simulink model "Grid_PBFORCAPF_ab_Detail_2013b_616"  (R2021b)
settings: Solver=FixedStepDiscrete  StartTime=0.0  StopTime=1.5  FixedStep=Ts_Power  RelTol=1e-3
InitFcn:
  | %% Sys Para
  | N=200;fg=50;Vbase=200;
  | Ts_Control=1/N/fg;
  | Tscon=Ts_Control;
  | Ts_Power=Ts_Control/128;
  | fsw=1/Ts_Control;
  | Vdcref=350;
  | Vdcini=Vdcref;
  | 
  | 
  | 
  | %% Load Side
  | Ll=2.0e-3;Rl=1e-2;
  | RL=100;
  | 
  | %% DG Circuit Parameters
  | %% LCL
  | L1_DG1=1.4e-3;R1=1e-3;
  | L2_DG1=0.4e-3;R2=1e-3;
  | Cx_DG1=6.3e-6;
  | 
  | L1_DG2=L1_DG1;L2_DG2=L2_DG1;Cx_DG2=Cx_DG1;
  | L1_DG3=L1_DG1;L2_DG3=L2_DG1;Cx_DG3=Cx_DG1;
  | Cdc=0.55e-3;
  | %PLL;
  | Kp_pll=88;
  | Ki_pll=0.4/Ts_Control;
  | 
  | %% DG2 Controller Parameters
  | Kpc_DG1=4.89;
  | Kic_DG1=0;
  | 
  | Kpdc_DG1=0.2;
  | Kidc_DG1=0.1;
undefined symbols (not defined in the file or in its folder): DiscIntNeverNeededParam, L2, Rd
libraries: spsThreePhaseSeriesRLCBranchLib x13, slpidlib x8, spsThreePhaseVIMeasurementLib x8, spsStairGeneratorLib x8, simulink x6, simulink_extras x6, spsSeriesRLCBranchLib x5, spsThreePhaseBreakerLib x5, spsUniversalBridgeLib x4, spsNeutralLib x4, spsGroundLib x3, spsPWMGenerator2LevelLib x3
(part 1 of 3)
Description:
  | Copyright 2008-2009 The MathWorks(TM), Inc.
settings Model: Creator=hyp01  LastModifiedBy=12586
settings SolverCC: MaxConsecutiveZCs=50000  AlgebraicLoopSolver=TrustRegion  SolverResetMethod=Robust
settings DataIOCC: SaveFormat=Array  SaveOutput=off  SaveTime=off  ReturnWorkspaceOutputs=off  SignalLoggingName=sigsOut
settings OptimizationCC: BlockReduction=off  BooleanDataType=off  ExpressionDepthLimit=2147483647  InitFltsAndDblsToZero=on  LifeSpan=inf
settings DebuggingCC: UnderspecifiedInitializationDetection=Classic  MergeDetectMultiDrivingBlocksExec=none  CheckExecutionContextPreStartOutputMsg=on  SignalResolutionControl=TryResolveAllWithWarning  MaxConsecutiveZCsMsg=none  MultiTaskDSMMsg=warning  MultiTaskCondExecSysMsg=none  FcnCallInpInsideContextMsg=warning  StateNameClashWarn=warning  SFUnexpectedBacktrackingDiag=warning  SFNoUnconditionalDefaultTransitionDiag=warning  SFExecutionAtInitializationDiag=none  SFMachineParentedDataDiag=warning  ArithmeticOperatorsInVariantConditions=warning
settings HardwareCC: ProdBitPerPointer=32  ProdBitPerSizeT=32  ProdBitPerPtrDiffT=32  ProdLargestAtomicFloat=None  ProdIntDivRoundTo=Undefined  ProdEndianess=Unspecified  ProdWordSize=32  ProdHWDeviceType=32-bit Generic  TargetBitPerPointer=64  TargetBitPerSizeT=64  TargetBitPerPtrDiffT=64  TargetLongLongMode=on  TargetIntDivRoundTo=Zero  TargetEndianess=LittleEndian  TargetWordSize=64  TargetHWDeviceType=MATLAB Host  ProdEqTarget=off
settings ModelReferenceCC: PropagateSignalLabelsOutOfModel=off
settings SFSimCC: SimUseLocalCustomCode=off  CustomCodeUndefinedFunction=UseInterfaceOnly
settings RTWCC: RTWUseLocalCustomCode=off  DLArmComputeVersion=20.02.1
settings CodeAppCC: StateflowObjectComments=on
settings GRTTargetCC: TargetFcnLib=ansi_tfl_tmw.mat  TargetLangStandard=C89/C90 (ANSI)  CombineOutputUpdateFcns=off  GRTInterface=on
settings ConfigComp: CovMetricSettings=dw  CovSaveCumulativeToWorkspaceVar=on  CovSaveSingleToWorkspaceVar=on  CovExternalEMLEnable=off
settings SimscapeCC: SimscapeNormalizeSystem=off

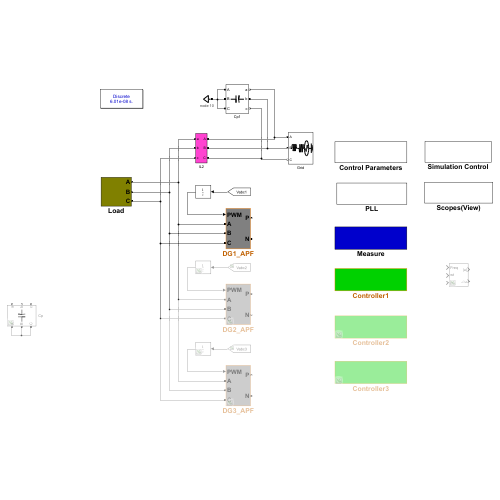
[thumbnail: Simulink's stored preview of the top-level diagram]
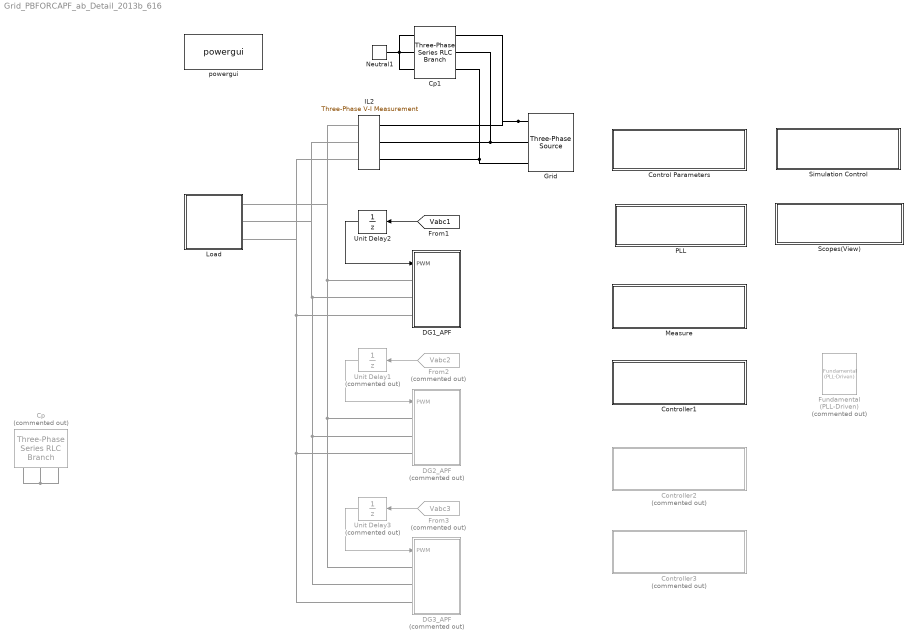
== system Grid_PBFORCAPF_ab_Detail_2013b_616 ==
  Control Parameters : Subsystem
  Controller1 : Subsystem
  Controller2 : Subsystem  Commented=on
  Controller3 : Subsystem  Commented=on
  Cp : spsThreePhaseSeriesRLCBranchLib/Three-Phase Series RLC Branch  Commented=on  LConnTagsString=A|B|C  RConnTagsString=A|B|C  BranchType=C  Resistance=Rd  Inductance=L2  Capacitance=22e-6  Measurements=Branch currents
  Cp1 : spsThreePhaseSeriesRLCBranchLib/Three-Phase Series RLC Branch  LConnTagsString=A|B|C  RConnTagsString=A|B|C  BranchType=C  Resistance=Rd  Inductance=L2  Capacitance=22e-6  Measurements=Branch currents
  DG1_APF : Subsystem
  DG2_APF : Subsystem  Commented=on
  DG3_APF : Subsystem  Commented=on
  From2 : From  Commented=on  GotoTag=Vabc2  TagVisibility=global
      settings: CloseFcn=tagdialog Close
  From3 : From  Commented=on  GotoTag=Vabc3  TagVisibility=global
      settings: CloseFcn=tagdialog Close
  Fundamental (PLL-Driven) : spsFundamentalPLLDrivenLib/Fundamental (PLL-Driven)  Commented=on  Finit=60  Fmin=45  InInit=[1, 0]  Ts=0
      settings: SourceProductBaseCode=PS
  Grid : spsThreePhaseSourceLib/Three-Phase Source  InternalConnection=Yg  VoltagePhases=off  Voltage=Vbase  PhaseAngle=-90  Voltage_phases=[380 380 380]/sqrt(3)  PhaseAngles_phases=[0 -120 +120]  Frequency=50  NonIdealSource=on  SpecifyImpedance=off  Resistance=0.5  Inductance=8e-3  ShortCircuitLevel=100e6  BaseVoltage=Vbase  XRratio=7  BusType=PV  Pref=10e3  Qref=0  Prefabc=[10e3, 10e3, 10e3]  Qrefabc=[0, 0, 0]  Qmin=-inf  Qmax=inf
  IL2 : spsThreePhaseVIMeasurementLib/Three-Phase V-I Measurement  VoltageMeasurement=phase-to-ground  SetLabelV=on  LabelV=Vpcc  Vpu=off  VpuLL=off  CurrentMeasurement=yes  SetLabelI=on  LabelI=Ig  Ipu=off  Pbase=100e6  Vbase=200  OutputType=Complex  PhasorSimulation=off  PSBequivalent=0
  Load : Subsystem
  Measure : Subsystem
  Neutral1 : spsNeutralLib/Neutral  LConnTagsString=a  NodeNumber=10
      settings: AttributesFormatString=node %<NodeNumber>  SourceProductBaseCode=PS
  PLL : Subsystem
  Scopes(View) : Subsystem
  Simulation Control : Subsystem
  Unit Delay1 : UnitDelay  Commented=on  SampleTime=Ts_Control  HasFrameUpgradeWarning=on
  Unit Delay2 : UnitDelay  SampleTime=Ts_Control  HasFrameUpgradeWarning=on
  Unit Delay3 : UnitDelay  Commented=on  SampleTime=Ts_Control  HasFrameUpgradeWarning=on
  powergui : spspowerguiLib/powergui  Priority=2  SimulationMode=Discrete  SampleTime=Ts_Power  frequency=60  Iterations=50  frequencyindice=0  Pbase=100e6  ErrMax=1e-4  UnitsV=kV  UnitsW=MW  buscounter=0  FunctionMessages=off  echomessages=on  EnableUseOfTLC=off  CurrentSourceSwitches=off  DisableSnubberDevices=off  DisableRonSwitches=off  DisableVfSwitches=off  DisplayEquations=off  AutomaticDiscreteSolvers=off  SolverType=Tustin/Backward Euler (TBE)  Interpol=off  ExternalGateDelay=off  methode=off  Ts=0  x0status=blocks  SPID=off  SwTol=0  HookPort=off  NonlinearTolerance=1e-4  nMaxIteration=100  ContinueOnMaxIteration=off  RestoreLinks=warning  ResistiveCurrentMeasurement=off  Frange=[0:2:500]  Ylog=off  Xlog=off  ShowGrid=off  save=off  variable=ZData  structure=AllData  ZoomFFT=on  StartTime=1.1  cycles=3  DisplayStyle=1  fundamental=50  FreqAxis=off  MaxFrequency=5000  frequencyindicesteady=1  RmsSteady=1  display=off
  wires:
  [Vabc1] -> Unit Delay2/1
  Unit Delay2/1 -> DG1_APF/1(PWM)
  From2/1 -> Unit Delay1/1
  From3/1 -> Unit Delay3/1
  Unit Delay3/1 -> DG3_APF/1(PWM)
  Unit Delay1/1 -> DG2_APF/1(PWM)
  connections:
  Grid/RConn1 -- IL2/LConn1 -- Cp1/RConn1
  Grid/RConn2 -- IL2/LConn2 -- Cp1/RConn2
  Cp1/LConn1 -- Cp1/LConn2 -- Cp1/LConn3 -- Neutral1/LConn1
  Cp/LConn1 -- Cp/LConn2 -- Cp/LConn3
  Cp1/RConn3 -- IL2/LConn3 -- Grid/RConn3
  DG3_APF/LConn1 -- DG1_APF/LConn1 -- IL2/RConn1 -- Load/LConn1 -- DG2_APF/LConn1
  DG2_APF/LConn2 -- DG3_APF/LConn2 -- DG1_APF/LConn2 -- IL2/RConn2 -- Load/LConn2
  DG3_APF/LConn3 -- DG1_APF/LConn3 -- IL2/RConn3 -- Load/LConn3 -- DG2_APF/LConn3

== system Grid_PBFORCAPF_ab_Detail_2013b_616/Control Parameters ==
  En_CVF_AD : Constant  Value=0.5  SampleTime=Tscon
  Fourier : spsFourierLib/Fourier  Commented=on  Freq=60  n=1  InInit=[0, 0]  Ts=0
      settings: SourceProductBaseCode=PS
  Goto2 : Goto  Commented=on  GotoTag=Leadk  TagVisibility=global
  Goto4 : Goto  Commented=on  GotoTag=Imref  TagVisibility=global
  Imref : Constant  Commented=on  Value=-5  SampleTime=Tscon
  Imref1 : Constant  Value=50  SampleTime=Tscon
  RSTTPLL : Constant  Value=0  SampleTime=Tscon
  SFIR : Constant  Commented=on  Value=2  SampleTime=Tscon
  tag scope: En_CVF_AD=global, RSTTPLL=global, fref=global
  wires:
  Imref/1 -> Goto4/1
  RSTTPLL/1 -> [RSTTPLL]
  En_CVF_AD/1 -> [En_CVF_AD]
  SFIR/1 -> Goto2/1
  Imref1/1 -> [fref]

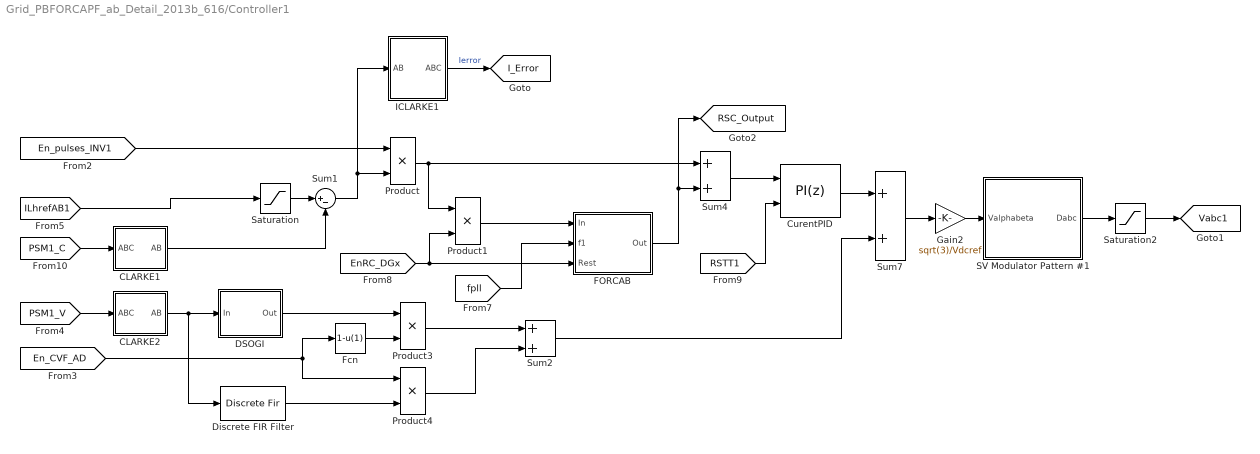
== system Grid_PBFORCAPF_ab_Detail_2013b_616/Controller1 ==
  CLARKE1 : Subsystem
  CLARKE2 : Subsystem
  "CurentPID " : slpidlib/PID Controller  Controller=PI  Form=Parallel  TimeDomain=Discrete-time  UseExternalTs=off  SampleTime=Ts_Control  IntegratorMethod=Backward Euler  FilterMethod=Forward Euler  ControllerParametersSource=internal  P=Kpc_DG1  I=Kic_DG1  D=0  N=100  UseFilter=on  TunerSelectOption=Transfer Function Based (PID Tuner App)  InitialConditionSource=internal  InitialConditionForIntegrator=0  InitialConditionForFilter=0  DifferentiatorICPrevScaledInput=0  ExternalReset=level  TrackingMode=off  Kt=1  LimitOutput=on  SatLimitsSource=internal  UpperSaturationLimit=700  LowerSaturationLimit=-700  LinearizeAsGain=off  AntiWindupMode=none  Kb=0.5  POutMin=[]  POutMax=[]  IOutMin=[]  IOutMax=[]  DOutMin=[]  DOutMax=[]  NOutMin=[]  NOutMax=[]  SumOutMin=[]  SumOutMax=[]  SaturationOutMin=[]  SaturationOutMax=[]  PParamMin=[]  PParamMax=[]  IParamMin=[]  IParamMax=[]  DParamMin=[]  DParamMax=[]  NParamMin=[]  NParamMax=[]  KbParamMin=[]  KbParamMax=[]  KtParamMin=[]  KtParamMax=[]  KbOutMin=[]  KbOutMax=[]  KtOutMin=[]  KtOutMax=[]  IntegratorOutMin=[]  IntegratorOutMax=[]  FilterOutMin=[]  FilterOutMax=[]  SumI1OutMin=[]  SumI1OutMax=[]  SumI2OutMin=[]  SumI2OutMax=[]  SumI3OutMin=[]  SumI3OutMax=[]  SumI4OutMin=[]  SumI4OutMax=[]  SumDOutMin=[]  SumDOutMax=[]  DifferentiatorOutMin=[]  DifferentiatorOutMax=[]  FilterDiffOutCoefMin=[]  FilterDiffOutCoefMax=[]  ReciprocalOutMin=[]  ReciprocalOutMax=[]  SumDenOutMin=[]  SumDenOutMax=[]  SumNumOutMin=[]  SumNumOutMax=[]  DivideOutMin=[]  DivideOutMax=[]  UdiffTsProdOutMin=[]  UdiffTsProdOutMax=[]  NTsProdOutMin=[]  NTsProdOutMax=[]  UintegralTsProdOutMin=[]  UintegralTsProdOutMax=[]  UngainTsProdOutMin=[]  UngainTsProdOutMax=[]  IntegratorContinuousStateAttributes=''  IntegratorStateMustResolveToSignalObject=off  IntegratorRTWStateStorageClass=Auto  FilterContinuousStateAttributes=''  FilterStateMustResolveToSignalObject=off  FilterRTWStateStorageClass=Auto  ParallelPVariant=InternalParameters  IdealPVariant=Disabled  IVariant=InternalParameters  DVariant=Disabled  IntegratorVariant=Discrete  SatVariant=Enabled  AWVariant=Passthrough  PCopyVariant=Disabled  TRVariant=Disabled  FdbkBlocksVariant=Forward  IdealPFdbkVariant=Disabled  SatFdbkVariant=Disabled  DerivativeFilterVariant=Disabled  NVariant=Disabled  NCopyVariant=Disabled_SignalSpec  FilterICVariant=Disabled  IntegratorICVariant=InternalICs  ExternalResetVariant=ExternalReset  TRSumVariant=Passthrough  SumFdbkVariant=Disabled  SumVariant=Sum_PI  TsampFilterVariant=InternalTs  TsampNgainVariant=Passthrough  TsampIntegralVariant=Passthrough  ExternalSaturationOutDataTypeStr=Inherit: Same as second input
  DSOGI : Subsystem  mask{h=1, KIh=31.4, wc=1, phch=0.09, Ts=Ts_Control}
      mask prompts: h "Harmonic order"; KIh "Integral KIh"; wc "Inversion maximum gains"; phch "phase compensation"; Ts "Sampling time"
  Discrete FIR Filter : DiscreteFir
  FORCAB : Subsystem  mask{Q=1, Lead=4, f2znum=0, f2zden=0, Ts=Ts_Control}
      mask prompts: Q "Damp factor"; Lead "Leading element d"; f2znum "num of compensation function Sz"; f2zden "den of compensation function Sz"; Ts "Sampling time"
      mask Display: disp('FORC')
  Fcn : Fcn  Expr=1-u(1)
  Gain2 : Gain  Gain=sqrt(3)/Vdcref
  ICLARKE1 : Subsystem
  Product{,1,3..4} (4 alike) : Product
  SV Modulator Pattern #1 : Subsystem  AncestorBlock=spsSVPWMGenerator2LevelModel/Continuous/SV Modulator Pattern #1
  Saturation : Saturate  UpperLimit=8  LowerLimit=-8
  Saturation2 : Saturate  UpperLimit=1  LowerLimit=0
  Sum1 : Sum  Inputs=|+-
  Sum2 : Sum
  Sum4 : Sum
  Sum7 : Sum
  tag scope: I_Error=global, RSC_Output=global, Vabc1=global
  wires:
  Product/1 -> Product1/1, Sum4/1
  [En_pulses_INV1] -> Product/1
  Sum1/1 -> ICLARKE1/1(AB), Product/2
  ICLARKE1/1(ABC) -> [I_Error]  "Ierror"
  Saturation/1 -> Sum1/1
  FORCAB/1(Out) -> [RSC_Output], Sum4/2
  [PSM1_V] -> CLARKE2/1(ABC)
  [RSTT1] -> "CurentPID "/2
  "CurentPID "/1 -> Sum7/1
  Sum7/1 -> Gain2/1
  Saturation2/1 -> [Vabc1]
  Product1/1 -> FORCAB/1(In)
  Gain2/1 -> SV Modulator Pattern #1/1(Valphabeta)
  SV Modulator Pattern #1/1(Dabc) -> Saturation2/1
  CLARKE2/1(AB) -> DSOGI/1(In), Discrete FIR Filter/1
  [EnRC_DGx] -> Product1/2, FORCAB/3(Rest)
  [PSM1_C] -> CLARKE1/1(ABC)
  CLARKE1/1(AB) -> Sum1/2
  DSOGI/1(Out) -> Product3/1
  Discrete FIR Filter/1 -> Product4/2
  [En_CVF_AD] -> Product4/1, Fcn/1
  Product3/1 -> Sum2/1
  Product4/1 -> Sum2/2
  Sum2/1 -> Sum7/2
  Fcn/1 -> Product3/2
  Sum4/1 -> "CurentPID "/1
  [ILhrefAB1] -> Saturation/1
  [fpll] -> FORCAB/2(f1)

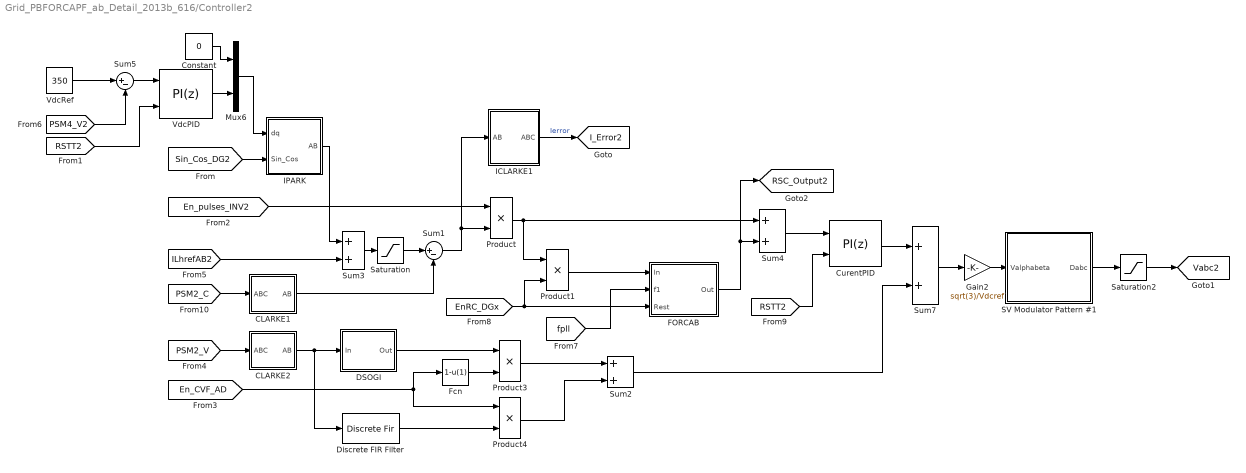
== system Grid_PBFORCAPF_ab_Detail_2013b_616/Controller2 ==
  CLARKE1 : Subsystem
  CLARKE2 : Subsystem
  Constant : Constant  Value=0  SampleTime=Tscon
  "CurentPID " : slpidlib/PID Controller  Controller=PI  Form=Parallel  TimeDomain=Discrete-time  UseExternalTs=off  SampleTime=Ts_Control  IntegratorMethod=Backward Euler  FilterMethod=Forward Euler  ControllerParametersSource=internal  P=Kpc_DG1  I=Kic_DG1  D=0  N=100  UseFilter=on  TunerSelectOption=Transfer Function Based (PID Tuner App)  InitialConditionSource=internal  InitialConditionForIntegrator=0  InitialConditionForFilter=0  DifferentiatorICPrevScaledInput=0  ExternalReset=level  TrackingMode=off  Kt=1  LimitOutput=on  SatLimitsSource=internal  UpperSaturationLimit=700  LowerSaturationLimit=-700  LinearizeAsGain=off  AntiWindupMode=none  Kb=0.5  POutMin=[]  POutMax=[]  IOutMin=[]  IOutMax=[]  DOutMin=[]  DOutMax=[]  NOutMin=[]  NOutMax=[]  SumOutMin=[]  SumOutMax=[]  SaturationOutMin=[]  SaturationOutMax=[]  PParamMin=[]  PParamMax=[]  IParamMin=[]  IParamMax=[]  DParamMin=[]  DParamMax=[]  NParamMin=[]  NParamMax=[]  KbParamMin=[]  KbParamMax=[]  KtParamMin=[]  KtParamMax=[]  KbOutMin=[]  KbOutMax=[]  KtOutMin=[]  KtOutMax=[]  IntegratorOutMin=[]  IntegratorOutMax=[]  FilterOutMin=[]  FilterOutMax=[]  SumI1OutMin=[]  SumI1OutMax=[]  SumI2OutMin=[]  SumI2OutMax=[]  SumI3OutMin=[]  SumI3OutMax=[]  SumI4OutMin=[]  SumI4OutMax=[]  SumDOutMin=[]  SumDOutMax=[]  DifferentiatorOutMin=[]  DifferentiatorOutMax=[]  FilterDiffOutCoefMin=[]  FilterDiffOutCoefMax=[]  ReciprocalOutMin=[]  ReciprocalOutMax=[]  SumDenOutMin=[]  SumDenOutMax=[]  SumNumOutMin=[]  SumNumOutMax=[]  DivideOutMin=[]  DivideOutMax=[]  UdiffTsProdOutMin=[]  UdiffTsProdOutMax=[]  NTsProdOutMin=[]  NTsProdOutMax=[]  UintegralTsProdOutMin=[]  UintegralTsProdOutMax=[]  UngainTsProdOutMin=[]  UngainTsProdOutMax=[]  IntegratorContinuousStateAttributes=''  IntegratorStateMustResolveToSignalObject=off  IntegratorRTWStateStorageClass=Auto  FilterContinuousStateAttributes=''  FilterStateMustResolveToSignalObject=off  FilterRTWStateStorageClass=Auto  ParallelPVariant=InternalParameters  IdealPVariant=Disabled  IVariant=InternalParameters  DVariant=Disabled  IntegratorVariant=Discrete  SatVariant=Enabled  AWVariant=Passthrough  PCopyVariant=Disabled  TRVariant=Disabled  FdbkBlocksVariant=Forward  IdealPFdbkVariant=Disabled  SatFdbkVariant=Disabled  DerivativeFilterVariant=Disabled  NVariant=Disabled  NCopyVariant=Disabled_SignalSpec  FilterICVariant=Disabled  IntegratorICVariant=InternalICs  ExternalResetVariant=ExternalReset  TRSumVariant=Passthrough  SumFdbkVariant=Disabled  SumVariant=Sum_PI  TsampFilterVariant=InternalTs  TsampNgainVariant=Passthrough  TsampIntegralVariant=Passthrough  ExternalSaturationOutDataTypeStr=Inherit: Same as second input
  DSOGI : Subsystem  mask{h=1, KIh=31.4, wc=1, phch=0.09, Ts=Ts_Control}
      mask prompts: h "Harmonic order"; KIh "Integral KIh"; wc "Inversion maximum gains"; phch "phase compensation"; Ts "Sampling time"
  Discrete FIR Filter : DiscreteFir
  FORCAB : Subsystem  mask{Q=1, Lead=4, f2znum=0, f2zden=0, Ts=Ts_Control}
      mask prompts: Q "Damp factor"; Lead "Leading element d"; f2znum "num of compensation function Sz"; f2zden "den of compensation function Sz"; Ts "Sampling time"
      mask Display: disp('FORC')
  Fcn : Fcn  Expr=1-u(1)
  Gain2 : Gain  Gain=sqrt(3)/Vdcref
  ICLARKE1 : Subsystem
  IPARK : Subsystem
  Mux6 : Mux  Inputs=2
  Product{,1,3..4} (4 alike) : Product
  SV Modulator Pattern #1 : Subsystem  AncestorBlock=spsSVPWMGenerator2LevelModel/Continuous/SV Modulator Pattern #1
  Saturation : Saturate  UpperLimit=8  LowerLimit=-8
  Saturation2 : Saturate  UpperLimit=1  LowerLimit=0
  Sum1 : Sum  Inputs=|+-
  Sum{2..4,7} (4 alike) : Sum
  Sum5 : Sum  Inputs=|+-
  VdcPID : slpidlib/PID Controller  Controller=PI  Form=Parallel  TimeDomain=Discrete-time  UseExternalTs=off  SampleTime=Ts_Control  IntegratorMethod=Backward Euler  FilterMethod=Forward Euler  ControllerParametersSource=internal  P=Kpdc_DG1  I=Kidc_DG1  D=0  N=100  UseFilter=on  TunerSelectOption=Transfer Function Based (PID Tuner App)  InitialConditionSource=internal  InitialConditionForIntegrator=0  InitialConditionForFilter=0  DifferentiatorICPrevScaledInput=0  ExternalReset=level  TrackingMode=off  Kt=1  LimitOutput=on  SatLimitsSource=internal  UpperSaturationLimit=5  LowerSaturationLimit=-5  LinearizeAsGain=off  AntiWindupMode=none  Kb=0.5  POutMin=[]  POutMax=[]  IOutMin=[]  IOutMax=[]  DOutMin=[]  DOutMax=[]  NOutMin=[]  NOutMax=[]  SumOutMin=[]  SumOutMax=[]  SaturationOutMin=[]  SaturationOutMax=[]  PParamMin=[]  PParamMax=[]  IParamMin=[]  IParamMax=[]  DParamMin=[]  DParamMax=[]  NParamMin=[]  NParamMax=[]  KbParamMin=[]  KbParamMax=[]  KtParamMin=[]  KtParamMax=[]  KbOutMin=[]  KbOutMax=[]  KtOutMin=[]  KtOutMax=[]  IntegratorOutMin=[]  IntegratorOutMax=[]  FilterOutMin=[]  FilterOutMax=[]  SumI1OutMin=[]  SumI1OutMax=[]  SumI2OutMin=[]  SumI2OutMax=[]  SumI3OutMin=[]  SumI3OutMax=[]  SumI4OutMin=[]  SumI4OutMax=[]  SumDOutMin=[]  SumDOutMax=[]  DifferentiatorOutMin=[]  DifferentiatorOutMax=[]  FilterDiffOutCoefMin=[]  FilterDiffOutCoefMax=[]  ReciprocalOutMin=[]  ReciprocalOutMax=[]  SumDenOutMin=[]  SumDenOutMax=[]  SumNumOutMin=[]  SumNumOutMax=[]  DivideOutMin=[]  DivideOutMax=[]  UdiffTsProdOutMin=[]  UdiffTsProdOutMax=[]  NTsProdOutMin=[]  NTsProdOutMax=[]  UintegralTsProdOutMin=[]  UintegralTsProdOutMax=[]  UngainTsProdOutMin=[]  UngainTsProdOutMax=[]  IntegratorContinuousStateAttributes=''  IntegratorStateMustResolveToSignalObject=off  IntegratorRTWStateStorageClass=Auto  FilterContinuousStateAttributes=''  FilterStateMustResolveToSignalObject=off  FilterRTWStateStorageClass=Auto  ParallelPVariant=InternalParameters  IdealPVariant=Disabled  IVariant=InternalParameters  DVariant=Disabled  IntegratorVariant=Discrete  SatVariant=Enabled  AWVariant=Passthrough  PCopyVariant=Disabled  TRVariant=Disabled  FdbkBlocksVariant=Forward  IdealPFdbkVariant=Disabled  SatFdbkVariant=Disabled  DerivativeFilterVariant=Disabled  NVariant=Disabled  NCopyVariant=Disabled_SignalSpec  FilterICVariant=Disabled  IntegratorICVariant=InternalICs  ExternalResetVariant=ExternalReset  TRSumVariant=Passthrough  SumFdbkVariant=Disabled  SumVariant=Sum_PI  TsampFilterVariant=InternalTs  TsampNgainVariant=Passthrough  TsampIntegralVariant=Passthrough  ExternalSaturationOutDataTypeStr=Inherit: Same as second input
  VdcRef : Constant  Value=350  SampleTime=Tscon
  tag scope: I_Error2=global, RSC_Output2=global, Vabc2=global
  wires:
  [fpll] -> FORCAB/2(f1)
  VdcRef/1 -> Sum5/1
  VdcPID/1 -> Mux6/2
  [Sin_Cos_DG2] -> IPARK/2(Sin_Cos)
  IPARK/1(AB) -> Sum3/1
  Mux6/1 -> IPARK/1(dq)
  Constant/1 -> Mux6/1
  [PSM4_V2] -> Sum5/2
  Sum5/1 -> VdcPID/1
  Sum3/1 -> Saturation/1
  [RSTT2] -> VdcPID/2
  Sum4/1 -> "CurentPID "/1
  Fcn/1 -> Product3/2
  Sum2/1 -> Sum7/2
  Product4/1 -> Sum2/2
  Product3/1 -> Sum2/1
  [En_CVF_AD] -> Fcn/1, Product4/1
  Discrete FIR Filter/1 -> Product4/2
  DSOGI/1(Out) -> Product3/1
  CLARKE1/1(AB) -> Sum1/2
  [PSM2_C] -> CLARKE1/1(ABC)
  [EnRC_DGx] -> FORCAB/3(Rest), Product1/2
  CLARKE2/1(AB) -> Discrete FIR Filter/1, DSOGI/1(In)
  SV Modulator Pattern #1/1(Dabc) -> Saturation2/1
  Gain2/1 -> SV Modulator Pattern #1/1(Valphabeta)
  Product1/1 -> FORCAB/1(In)
  Saturation2/1 -> [Vabc2]
  Sum7/1 -> Gain2/1
  "CurentPID "/1 -> Sum7/1
  [RSTT2] -> "CurentPID "/2
  [PSM2_V] -> CLARKE2/1(ABC)
  FORCAB/1(Out) -> Sum4/2, [RSC_Output2]
  Saturation/1 -> Sum1/1
  ICLARKE1/1(ABC) -> [I_Error2]  "Ierror"
  Sum1/1 -> Product/2, ICLARKE1/1(AB)
  [En_pulses_INV2] -> Product/1
  [ILhrefAB2] -> Sum3/2
  Product/1 -> Sum4/1, Product1/1

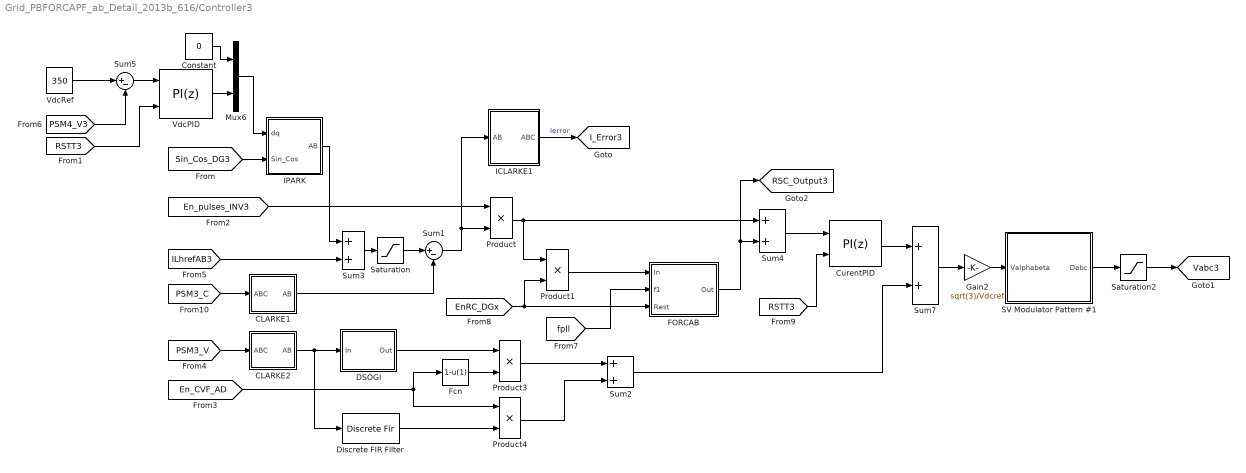
== system Grid_PBFORCAPF_ab_Detail_2013b_616/Controller3 ==
  CLARKE1 : Subsystem
  CLARKE2 : Subsystem
  Constant : Constant  Value=0  SampleTime=Tscon
  "CurentPID " : slpidlib/PID Controller  Controller=PI  Form=Parallel  TimeDomain=Discrete-time  UseExternalTs=off  SampleTime=Ts_Control  IntegratorMethod=Backward Euler  FilterMethod=Forward Euler  ControllerParametersSource=internal  P=Kpc_DG1  I=Kic_DG1  D=0  N=100  UseFilter=on  TunerSelectOption=Transfer Function Based (PID Tuner App)  InitialConditionSource=internal  InitialConditionForIntegrator=0  InitialConditionForFilter=0  DifferentiatorICPrevScaledInput=0  ExternalReset=level  TrackingMode=off  Kt=1  LimitOutput=on  SatLimitsSource=internal  UpperSaturationLimit=700  LowerSaturationLimit=-700  LinearizeAsGain=off  AntiWindupMode=none  Kb=0.5  POutMin=[]  POutMax=[]  IOutMin=[]  IOutMax=[]  DOutMin=[]  DOutMax=[]  NOutMin=[]  NOutMax=[]  SumOutMin=[]  SumOutMax=[]  SaturationOutMin=[]  SaturationOutMax=[]  PParamMin=[]  PParamMax=[]  IParamMin=[]  IParamMax=[]  DParamMin=[]  DParamMax=[]  NParamMin=[]  NParamMax=[]  KbParamMin=[]  KbParamMax=[]  KtParamMin=[]  KtParamMax=[]  KbOutMin=[]  KbOutMax=[]  KtOutMin=[]  KtOutMax=[]  IntegratorOutMin=[]  IntegratorOutMax=[]  FilterOutMin=[]  FilterOutMax=[]  SumI1OutMin=[]  SumI1OutMax=[]  SumI2OutMin=[]  SumI2OutMax=[]  SumI3OutMin=[]  SumI3OutMax=[]  SumI4OutMin=[]  SumI4OutMax=[]  SumDOutMin=[]  SumDOutMax=[]  DifferentiatorOutMin=[]  DifferentiatorOutMax=[]  FilterDiffOutCoefMin=[]  FilterDiffOutCoefMax=[]  ReciprocalOutMin=[]  ReciprocalOutMax=[]  SumDenOutMin=[]  SumDenOutMax=[]  SumNumOutMin=[]  SumNumOutMax=[]  DivideOutMin=[]  DivideOutMax=[]  UdiffTsProdOutMin=[]  UdiffTsProdOutMax=[]  NTsProdOutMin=[]  NTsProdOutMax=[]  UintegralTsProdOutMin=[]  UintegralTsProdOutMax=[]  UngainTsProdOutMin=[]  UngainTsProdOutMax=[]  IntegratorContinuousStateAttributes=''  IntegratorStateMustResolveToSignalObject=off  IntegratorRTWStateStorageClass=Auto  FilterContinuousStateAttributes=''  FilterStateMustResolveToSignalObject=off  FilterRTWStateStorageClass=Auto  ParallelPVariant=InternalParameters  IdealPVariant=Disabled  IVariant=InternalParameters  DVariant=Disabled  IntegratorVariant=Discrete  SatVariant=Enabled  AWVariant=Passthrough  PCopyVariant=Disabled  TRVariant=Disabled  FdbkBlocksVariant=Forward  IdealPFdbkVariant=Disabled  SatFdbkVariant=Disabled  DerivativeFilterVariant=Disabled  NVariant=Disabled  NCopyVariant=Disabled_SignalSpec  FilterICVariant=Disabled  IntegratorICVariant=InternalICs  ExternalResetVariant=ExternalReset  TRSumVariant=Passthrough  SumFdbkVariant=Disabled  SumVariant=Sum_PI  TsampFilterVariant=InternalTs  TsampNgainVariant=Passthrough  TsampIntegralVariant=Passthrough  ExternalSaturationOutDataTypeStr=Inherit: Same as second input
  DSOGI : Subsystem  mask{h=1, KIh=31.4, wc=1, phch=0.09, Ts=Ts_Control}
      mask prompts: h "Harmonic order"; KIh "Integral KIh"; wc "Inversion maximum gains"; phch "phase compensation"; Ts "Sampling time"
  Discrete FIR Filter : DiscreteFir
  FORCAB : Subsystem  mask{Q=1, Lead=4, f2znum=0, f2zden=0, Ts=Ts_Control}
      mask prompts: Q "Damp factor"; Lead "Leading element d"; f2znum "num of compensation function Sz"; f2zden "den of compensation function Sz"; Ts "Sampling time"
      mask Display: disp('FORC')
  Fcn : Fcn  Expr=1-u(1)
  Gain2 : Gain  Gain=sqrt(3)/Vdcref
  ICLARKE1 : Subsystem
  IPARK : Subsystem
  Mux6 : Mux  Inputs=2
  Product{,1,3..4} (4 alike) : Product
  SV Modulator Pattern #1 : Subsystem  AncestorBlock=spsSVPWMGenerator2LevelModel/Continuous/SV Modulator Pattern #1
  Saturation : Saturate  UpperLimit=8  LowerLimit=-8
  Saturation2 : Saturate  UpperLimit=1  LowerLimit=0
  Sum1 : Sum  Inputs=|+-
  Sum{2..4,7} (4 alike) : Sum
  Sum5 : Sum  Inputs=|+-
  VdcPID : slpidlib/PID Controller  Controller=PI  Form=Parallel  TimeDomain=Discrete-time  UseExternalTs=off  SampleTime=Ts_Control  IntegratorMethod=Backward Euler  FilterMethod=Forward Euler  ControllerParametersSource=internal  P=Kpdc_DG1  I=Kidc_DG1  D=0  N=100  UseFilter=on  TunerSelectOption=Transfer Function Based (PID Tuner App)  InitialConditionSource=internal  InitialConditionForIntegrator=0  InitialConditionForFilter=0  DifferentiatorICPrevScaledInput=0  ExternalReset=level  TrackingMode=off  Kt=1  LimitOutput=on  SatLimitsSource=internal  UpperSaturationLimit=5  LowerSaturationLimit=-5  LinearizeAsGain=off  AntiWindupMode=none  Kb=0.5  POutMin=[]  POutMax=[]  IOutMin=[]  IOutMax=[]  DOutMin=[]  DOutMax=[]  NOutMin=[]  NOutMax=[]  SumOutMin=[]  SumOutMax=[]  SaturationOutMin=[]  SaturationOutMax=[]  PParamMin=[]  PParamMax=[]  IParamMin=[]  IParamMax=[]  DParamMin=[]  DParamMax=[]  NParamMin=[]  NParamMax=[]  KbParamMin=[]  KbParamMax=[]  KtParamMin=[]  KtParamMax=[]  KbOutMin=[]  KbOutMax=[]  KtOutMin=[]  KtOutMax=[]  IntegratorOutMin=[]  IntegratorOutMax=[]  FilterOutMin=[]  FilterOutMax=[]  SumI1OutMin=[]  SumI1OutMax=[]  SumI2OutMin=[]  SumI2OutMax=[]  SumI3OutMin=[]  SumI3OutMax=[]  SumI4OutMin=[]  SumI4OutMax=[]  SumDOutMin=[]  SumDOutMax=[]  DifferentiatorOutMin=[]  DifferentiatorOutMax=[]  FilterDiffOutCoefMin=[]  FilterDiffOutCoefMax=[]  ReciprocalOutMin=[]  ReciprocalOutMax=[]  SumDenOutMin=[]  SumDenOutMax=[]  SumNumOutMin=[]  SumNumOutMax=[]  DivideOutMin=[]  DivideOutMax=[]  UdiffTsProdOutMin=[]  UdiffTsProdOutMax=[]  NTsProdOutMin=[]  NTsProdOutMax=[]  UintegralTsProdOutMin=[]  UintegralTsProdOutMax=[]  UngainTsProdOutMin=[]  UngainTsProdOutMax=[]  IntegratorContinuousStateAttributes=''  IntegratorStateMustResolveToSignalObject=off  IntegratorRTWStateStorageClass=Auto  FilterContinuousStateAttributes=''  FilterStateMustResolveToSignalObject=off  FilterRTWStateStorageClass=Auto  ParallelPVariant=InternalParameters  IdealPVariant=Disabled  IVariant=InternalParameters  DVariant=Disabled  IntegratorVariant=Discrete  SatVariant=Enabled  AWVariant=Passthrough  PCopyVariant=Disabled  TRVariant=Disabled  FdbkBlocksVariant=Forward  IdealPFdbkVariant=Disabled  SatFdbkVariant=Disabled  DerivativeFilterVariant=Disabled  NVariant=Disabled  NCopyVariant=Disabled_SignalSpec  FilterICVariant=Disabled  IntegratorICVariant=InternalICs  ExternalResetVariant=ExternalReset  TRSumVariant=Passthrough  SumFdbkVariant=Disabled  SumVariant=Sum_PI  TsampFilterVariant=InternalTs  TsampNgainVariant=Passthrough  TsampIntegralVariant=Passthrough  ExternalSaturationOutDataTypeStr=Inherit: Same as second input
  VdcRef : Constant  Value=350  SampleTime=Tscon
  tag scope: I_Error3=global, RSC_Output3=global, Vabc3=global
  wires:
  Product/1 -> Product1/1, Sum4/1
  [ILhrefAB3] -> Sum3/2
  [En_pulses_INV3] -> Product/1
  Sum1/1 -> ICLARKE1/1(AB), Product/2
  ICLARKE1/1(ABC) -> [I_Error3]  "Ierror"
  Saturation/1 -> Sum1/1
  FORCAB/1(Out) -> [RSC_Output3], Sum4/2
  [PSM3_V] -> CLARKE2/1(ABC)
  [RSTT3] -> "CurentPID "/2
  "CurentPID "/1 -> Sum7/1
  Sum7/1 -> Gain2/1
  Saturation2/1 -> [Vabc3]
  Product1/1 -> FORCAB/1(In)
  Gain2/1 -> SV Modulator Pattern #1/1(Valphabeta)
  SV Modulator Pattern #1/1(Dabc) -> Saturation2/1
  CLARKE2/1(AB) -> DSOGI/1(In), Discrete FIR Filter/1
  [EnRC_DGx] -> Product1/2, FORCAB/3(Rest)
  [PSM3_C] -> CLARKE1/1(ABC)
  CLARKE1/1(AB) -> Sum1/2
  DSOGI/1(Out) -> Product3/1
  Discrete FIR Filter/1 -> Product4/2
  [En_CVF_AD] -> Product4/1, Fcn/1
  Product3/1 -> Sum2/1
  Product4/1 -> Sum2/2
  Sum2/1 -> Sum7/2
  Fcn/1 -> Product3/2
  Sum4/1 -> "CurentPID "/1
  [RSTT3] -> VdcPID/2
  Sum3/1 -> Saturation/1
  Sum5/1 -> VdcPID/1
  [PSM4_V3] -> Sum5/2
  Constant/1 -> Mux6/1
  Mux6/1 -> IPARK/1(dq)
  IPARK/1(AB) -> Sum3/1
  [Sin_Cos_DG3] -> IPARK/2(Sin_Cos)
  VdcPID/1 -> Mux6/2
  VdcRef/1 -> Sum5/1
  [fpll] -> FORCAB/2(f1)

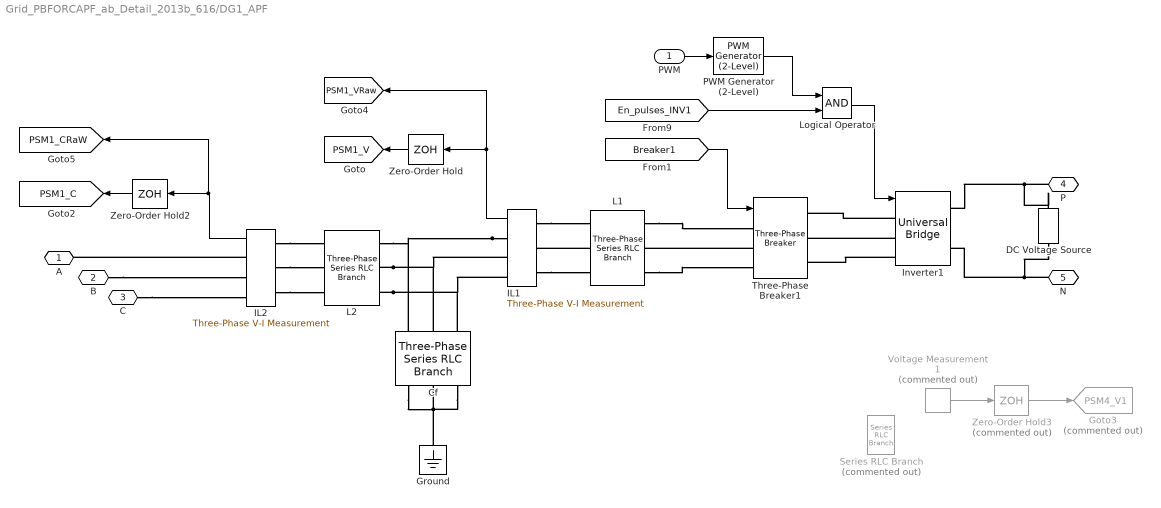
== system Grid_PBFORCAPF_ab_Detail_2013b_616/DG1_APF ==
  PWM : Inport
  Cf : spsThreePhaseSeriesRLCBranchLib/Three-Phase Series RLC Branch  LConnTagsString=A|B|C  RConnTagsString=A|B|C  BranchType=C  Resistance=Rd  Inductance=L2  Capacitance=Cx_DG1  Measurements=None
  DC Voltage Source : spsDCVoltageSourceLib/DC Voltage Source  Amplitude=350  Measurements=None
  Goto3 : Goto  Commented=on  GotoTag=PSM4_V1  TagVisibility=global
  Ground : spsGroundLib/Ground  LConnTagsString=a
  IL1 : spsThreePhaseVIMeasurementLib/Three-Phase V-I Measurement  VoltageMeasurement=phase-to-ground  SetLabelV=off  LabelV=Vc1  Vpu=off  VpuLL=off  CurrentMeasurement=no  SetLabelI=off  LabelI=IL1  Ipu=off  Pbase=100e6  Vbase=280  OutputType=Complex  PhasorSimulation=off  PSBequivalent=0
  IL2 : spsThreePhaseVIMeasurementLib/Three-Phase V-I Measurement  VoltageMeasurement=no  SetLabelV=off  LabelV=Vabc  Vpu=off  VpuLL=off  CurrentMeasurement=yes  SetLabelI=off  LabelI=IO1  Ipu=off  Pbase=100e6  Vbase=280  OutputType=Complex  PhasorSimulation=off  PSBequivalent=0
  Inverter1 : spsUniversalBridgeLib/Universal Bridge  Arms=3  SnubberResistance=1e5  SnubberCapacitance=inf  Device=IGBT / Diodes  Ron=1e-3  Lon=0  ForwardVoltages="[  0  0  ]"  ForwardVoltage=0  GTOparameters=[ 10e-6 , 20e-6 ]  IGBTparameters=[ 1e-6 , 2e-6 ]  Measurements=None  Measurements_2=None  converterType=Rectifier
  L1 : spsThreePhaseSeriesRLCBranchLib/Three-Phase Series RLC Branch  LConnTagsString=A|B|C  RConnTagsString=A|B|C  BranchType=RL  Resistance=R1  Inductance=L1_DG1  Capacitance=1e-6  Measurements=Branch currents
  L2 : spsThreePhaseSeriesRLCBranchLib/Three-Phase Series RLC Branch  LConnTagsString=A|B|C  RConnTagsString=A|B|C  BranchType=RL  Resistance=R2  Inductance=L2_DG2  Capacitance=1e-6  Measurements=Branch currents
  Logical Operator : Logic  AllPortsSameDT=off  OutDataTypeStr=boolean
  PWM Generator (2-Level) : spsPWMGenerator2LevelLib/PWM Generator (2-Level)  ModulatorType=Three-phase bridge (6 pulses)  ModulatorMode=Unsynchronized  Fc=fsw  Pc=0  nF=27  MinMax=[0 1]  SamplingTechnique=Symmetrical regular (single edge)  ModulatingSignals=off  m=0.8  Freq=60  Phase=0  Ts=Ts_Power  ShowCarrierOutport=off
  Series RLC Branch : spsSeriesRLCBranchLib/Series RLC Branch  Commented=on  LConnTagsString=__new0  RConnTagsString=__new0  BranchType=C  Resistance=0.01  Inductance=1e-3  SetiL0=off  InitialCurrent=0  Capacitance=Cdc  Setx0=on  InitialVoltage=Vdcini  Measurements=None
  Three-Phase Breaker1 : spsThreePhaseBreakerLib/Three-Phase Breaker  InitialState=open  SwitchA=on  SwitchB=on  SwitchC=on  SwitchTimes="[1/60  5/60]"  External=on  BreakerResistance=0.01  SnubberResistance=1e6  SnubberCapacitance=inf  Measurements=None
  Voltage Measurement1 : spsVoltageMeasurementLib/Voltage Measurement  Commented=on  PhasorSimulation=off  OutputType=Complex  PSBequivalent=0
  Zero-Order Hold : ZeroOrderHold  SampleTime=Ts_Control
  Zero-Order Hold2 : ZeroOrderHold  SampleTime=Ts_Control
  Zero-Order Hold3 : ZeroOrderHold  Commented=on  SampleTime=Ts_Control
  A : PMIOPort  Side=Left
  B : PMIOPort  Port=2  Side=Left
  C : PMIOPort  Port=3  Side=Left
  P : PMIOPort  Port=4  Side=Right
  N : PMIOPort  Port=5  Side=Right
  tag scope: PSM1_C=global, PSM1_CRaW=global, PSM1_V=global, PSM1_VRaw=global
  wires:
  IL2/1 -> [PSM1_CRaW], Zero-Order Hold2/1
  Zero-Order Hold2/1 -> [PSM1_C]
  Zero-Order Hold/1 -> [PSM1_V]
  IL1/1 -> [PSM1_VRaw], Zero-Order Hold/1
  [Breaker1] -> Three-Phase Breaker1/1
  [En_pulses_INV1] -> Logical Operator/2
  Logical Operator/1 -> Inverter1/1
  PWM/1 -> PWM Generator (2-Level)/1
  PWM Generator (2-Level)/1 -> Logical Operator/1
  Zero-Order Hold3/1 -> Goto3/1
  Voltage Measurement1/1 -> Zero-Order Hold3/1
  connections:
  IL2/RConn1 -- A/RConn1
  C/RConn1 -- IL2/RConn3
  B/RConn1 -- IL2/RConn2
  IL1/LConn3 -- L1/LConn3
  L1/LConn2 -- IL1/LConn2
  IL1/LConn1 -- L1/LConn1
  IL2/LConn3 -- L2/LConn3
  IL2/LConn2 -- L2/LConn2
  IL2/LConn1 -- L2/LConn1
  Cf/LConn3 -- Ground/LConn1 -- Cf/LConn1 -- Cf/LConn2
  L2/RConn3 -- Cf/RConn3 -- IL1/RConn3
  L2/RConn2 -- Cf/RConn2 -- IL1/RConn2
  IL1/RConn1 -- Cf/RConn1 -- L2/RConn1
  N/RConn1 -- Inverter1/RConn2 -- DC Voltage Source/LConn1
  P/RConn1 -- Inverter1/RConn1 -- DC Voltage Source/RConn1
  Three-Phase Breaker1/LConn2 -- L1/RConn2
  L1/RConn1 -- Three-Phase Breaker1/LConn1
  L1/RConn3 -- Three-Phase Breaker1/LConn3
  Inverter1/LConn2 -- Three-Phase Breaker1/RConn2
  Inverter1/LConn3 -- Three-Phase Breaker1/RConn3
  Inverter1/LConn1 -- Three-Phase Breaker1/RConn1

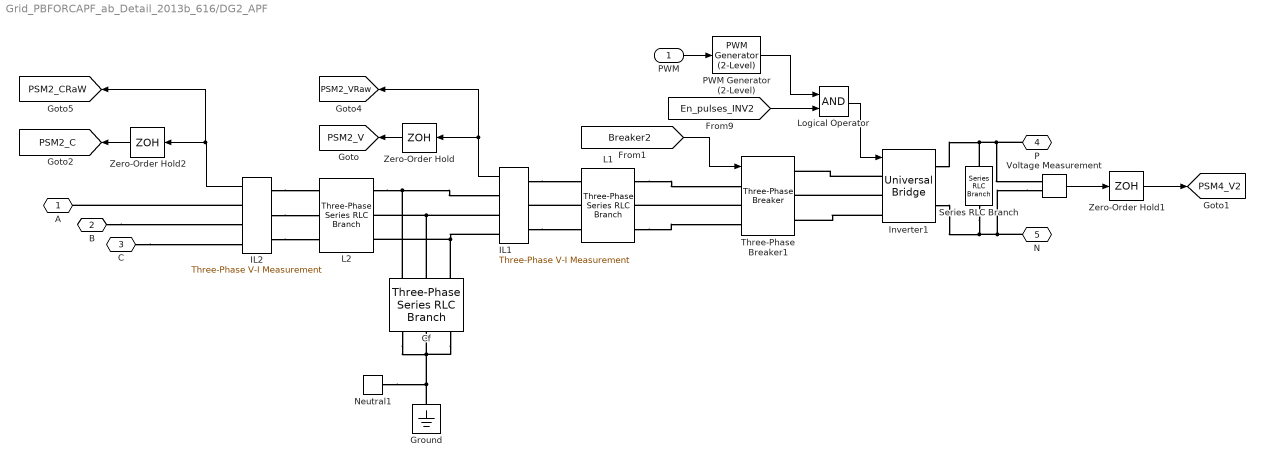
== system Grid_PBFORCAPF_ab_Detail_2013b_616/DG2_APF ==
  PWM : Inport
  Cf : spsThreePhaseSeriesRLCBranchLib/Three-Phase Series RLC Branch  LConnTagsString=A|B|C  RConnTagsString=A|B|C  BranchType=C  Resistance=Rd  Inductance=L2  Capacitance=Cx_DG2  Measurements=None
  Ground : spsGroundLib/Ground  LConnTagsString=a
  IL1 : spsThreePhaseVIMeasurementLib/Three-Phase V-I Measurement  VoltageMeasurement=phase-to-ground  SetLabelV=off  LabelV=Vc1  Vpu=off  VpuLL=off  CurrentMeasurement=no  SetLabelI=off  LabelI=IL1  Ipu=off  Pbase=100e6  Vbase=280  OutputType=Complex  PhasorSimulation=off  PSBequivalent=0
  IL2 : spsThreePhaseVIMeasurementLib/Three-Phase V-I Measurement  VoltageMeasurement=no  SetLabelV=on  LabelV=Vs2abc  Vpu=on  VpuLL=off  CurrentMeasurement=yes  SetLabelI=off  LabelI=IO1  Ipu=off  Pbase=100e6  Vbase=280  OutputType=Complex  PhasorSimulation=off  PSBequivalent=0
  Inverter1 : spsUniversalBridgeLib/Universal Bridge  Arms=3  SnubberResistance=1e5  SnubberCapacitance=inf  Device=IGBT / Diodes  Ron=1e-3  Lon=0  ForwardVoltages="[  0  0  ]"  ForwardVoltage=0  GTOparameters=[ 10e-6 , 20e-6 ]  IGBTparameters=[ 1e-6 , 2e-6 ]  Measurements=None  Measurements_2=None  converterType=Rectifier
  L1 : spsThreePhaseSeriesRLCBranchLib/Three-Phase Series RLC Branch  LConnTagsString=A|B|C  RConnTagsString=A|B|C  BranchType=RL  Resistance=R1  Inductance=L1_DG2  Capacitance=1e-6  Measurements=Branch currents
  L2 : spsThreePhaseSeriesRLCBranchLib/Three-Phase Series RLC Branch  LConnTagsString=A|B|C  RConnTagsString=A|B|C  BranchType=RL  Resistance=R2  Inductance=L2_DG2  Capacitance=1e-6  Measurements=Branch currents
  Logical Operator : Logic  AllPortsSameDT=off  OutDataTypeStr=boolean
  Neutral1 : spsNeutralLib/Neutral  LConnTagsString=a  NodeNumber=10
      settings: AttributesFormatString=node %<NodeNumber>  SourceProductBaseCode=PS
  PWM Generator (2-Level) : spsPWMGenerator2LevelLib/PWM Generator (2-Level)  ModulatorType=Three-phase bridge (6 pulses)  ModulatorMode=Unsynchronized  Fc=fsw  Pc=0  nF=27  MinMax=[0 1]  SamplingTechnique=Symmetrical regular (single edge)  ModulatingSignals=off  m=0.8  Freq=60  Phase=0  Ts=Ts_Power  ShowCarrierOutport=off
  Series RLC Branch : spsSeriesRLCBranchLib/Series RLC Branch  LConnTagsString=__new0  RConnTagsString=__new0  BranchType=C  Resistance=0.01  Inductance=1e-3  SetiL0=off  InitialCurrent=0  Capacitance=Cdc  Setx0=on  InitialVoltage=Vdcini  Measurements=None
  Three-Phase Breaker1 : spsThreePhaseBreakerLib/Three-Phase Breaker  InitialState=open  SwitchA=on  SwitchB=on  SwitchC=on  SwitchTimes="[1/60  5/60]"  External=on  BreakerResistance=0.01  SnubberResistance=1e6  SnubberCapacitance=inf  Measurements=None
  Voltage Measurement : spsVoltageMeasurementLib/Voltage Measurement  PhasorSimulation=off  OutputType=Complex  PSBequivalent=0
  Zero-Order Hold : ZeroOrderHold  SampleTime=Ts_Control
  Zero-Order Hold1 : ZeroOrderHold  SampleTime=Ts_Control
  Zero-Order Hold2 : ZeroOrderHold  SampleTime=Ts_Control
  A : PMIOPort  Side=Left
  B : PMIOPort  Port=2  Side=Left
  C : PMIOPort  Port=3  Side=Left
  P : PMIOPort  Port=4  Side=Right
  N : PMIOPort  Port=5  Side=Right
  tag scope: PSM2_C=global, PSM2_CRaW=global, PSM2_V=global, PSM2_VRaw=global, PSM4_V2=global
  wires:
  PWM Generator (2-Level)/1 -> Logical Operator/1
  PWM/1 -> PWM Generator (2-Level)/1
  Logical Operator/1 -> Inverter1/1
  [En_pulses_INV2] -> Logical Operator/2
  [Breaker2] -> Three-Phase Breaker1/1
  IL1/1 -> Zero-Order Hold/1, [PSM2_VRaw]
  Zero-Order Hold/1 -> [PSM2_V]
  Zero-Order Hold2/1 -> [PSM2_C]
  IL2/1 -> Zero-Order Hold2/1, [PSM2_CRaW]
  Voltage Measurement/1 -> Zero-Order Hold1/1
  Zero-Order Hold1/1 -> [PSM4_V2]
  connections:
  Inverter1/LConn1 -- Three-Phase Breaker1/RConn1
  Inverter1/LConn3 -- Three-Phase Breaker1/RConn3
  Inverter1/LConn2 -- Three-Phase Breaker1/RConn2
  L1/RConn3 -- Three-Phase Breaker1/LConn3
  L1/RConn1 -- Three-Phase Breaker1/LConn1
  Three-Phase Breaker1/LConn2 -- L1/RConn2
  L2/RConn1 -- IL1/RConn1 -- Cf/RConn1
  IL1/RConn2 -- Cf/RConn2 -- L2/RConn2
  IL1/RConn3 -- Cf/RConn3 -- L2/RConn3
  Cf/LConn2 -- Cf/LConn1 -- Ground/LConn1 -- Neutral1/LConn1 -- Cf/LConn3
  IL2/LConn1 -- L2/LConn1
  IL2/LConn2 -- L2/LConn2
  IL2/LConn3 -- L2/LConn3
  IL1/LConn1 -- L1/LConn1
  L1/LConn2 -- IL1/LConn2
  IL1/LConn3 -- L1/LConn3
  B/RConn1 -- IL2/RConn2
  C/RConn1 -- IL2/RConn3
  IL2/RConn1 -- A/RConn1
  Voltage Measurement/LConn2 -- N/RConn1 -- Inverter1/RConn2 -- Series RLC Branch/RConn1
  Series RLC Branch/LConn1 -- Inverter1/RConn1 -- P/RConn1 -- Voltage Measurement/LConn1

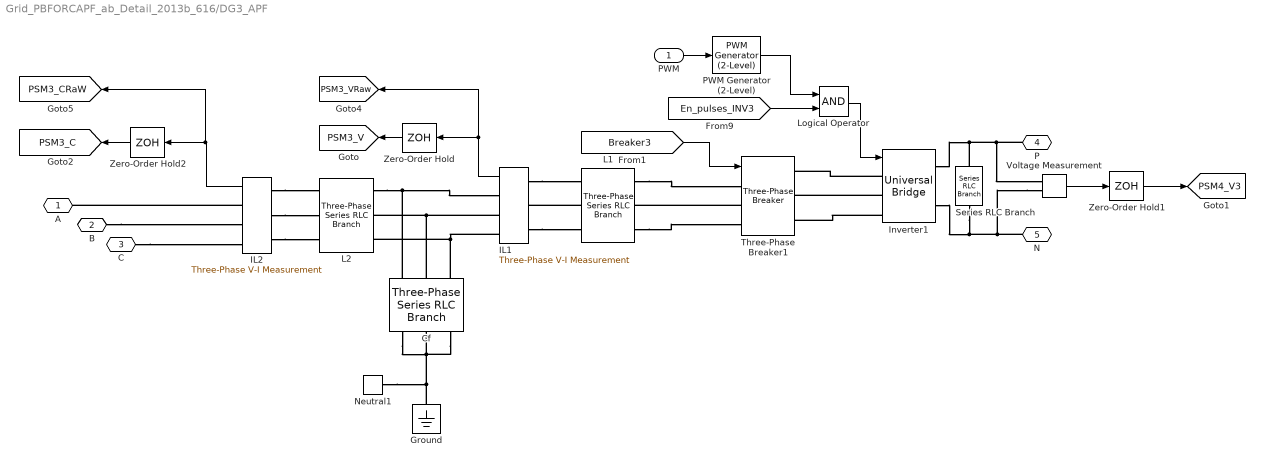
== system Grid_PBFORCAPF_ab_Detail_2013b_616/DG3_APF ==
  PWM : Inport
  Cf : spsThreePhaseSeriesRLCBranchLib/Three-Phase Series RLC Branch  LConnTagsString=A|B|C  RConnTagsString=A|B|C  BranchType=C  Resistance=Rd  Inductance=L2  Capacitance=Cx_DG3  Measurements=None
  Ground : spsGroundLib/Ground  LConnTagsString=a
  IL1 : spsThreePhaseVIMeasurementLib/Three-Phase V-I Measurement  VoltageMeasurement=phase-to-ground  SetLabelV=off  LabelV=Vc1  Vpu=off  VpuLL=off  CurrentMeasurement=no  SetLabelI=off  LabelI=IL1  Ipu=off  Pbase=100e6  Vbase=280  OutputType=Complex  PhasorSimulation=off  PSBequivalent=0
  IL2 : spsThreePhaseVIMeasurementLib/Three-Phase V-I Measurement  VoltageMeasurement=no  SetLabelV=on  LabelV=Vs2abc  Vpu=on  VpuLL=off  CurrentMeasurement=yes  SetLabelI=off  LabelI=IO1  Ipu=off  Pbase=100e6  Vbase=280  OutputType=Complex  PhasorSimulation=off  PSBequivalent=0
  Inverter1 : spsUniversalBridgeLib/Universal Bridge  Arms=3  SnubberResistance=1e5  SnubberCapacitance=inf  Device=IGBT / Diodes  Ron=1e-3  Lon=0  ForwardVoltages="[  0  0  ]"  ForwardVoltage=0  GTOparameters=[ 10e-6 , 20e-6 ]  IGBTparameters=[ 1e-6 , 2e-6 ]  Measurements=None  Measurements_2=None  converterType=Rectifier
  L1 : spsThreePhaseSeriesRLCBranchLib/Three-Phase Series RLC Branch  LConnTagsString=A|B|C  RConnTagsString=A|B|C  BranchType=RL  Resistance=R1  Inductance=L1_DG3  Capacitance=1e-6  Measurements=Branch currents
  L2 : spsThreePhaseSeriesRLCBranchLib/Three-Phase Series RLC Branch  LConnTagsString=A|B|C  RConnTagsString=A|B|C  BranchType=RL  Resistance=R2  Inductance=L2_DG3  Capacitance=1e-6  Measurements=Branch currents
  Logical Operator : Logic  AllPortsSameDT=off  OutDataTypeStr=boolean
  Neutral1 : spsNeutralLib/Neutral  LConnTagsString=a  NodeNumber=10
      settings: AttributesFormatString=node %<NodeNumber>  SourceProductBaseCode=PS
  PWM Generator (2-Level) : spsPWMGenerator2LevelLib/PWM Generator (2-Level)  ModulatorType=Three-phase bridge (6 pulses)  ModulatorMode=Unsynchronized  Fc=fsw  Pc=0  nF=27  MinMax=[0 1]  SamplingTechnique=Symmetrical regular (single edge)  ModulatingSignals=off  m=0.8  Freq=60  Phase=0  Ts=Ts_Power  ShowCarrierOutport=off
  Series RLC Branch : spsSeriesRLCBranchLib/Series RLC Branch  LConnTagsString=__new0  RConnTagsString=__new0  BranchType=C  Resistance=0.01  Inductance=1e-3  SetiL0=off  InitialCurrent=0  Capacitance=Cdc  Setx0=on  InitialVoltage=Vdcini  Measurements=None
  Three-Phase Breaker1 : spsThreePhaseBreakerLib/Three-Phase Breaker  InitialState=open  SwitchA=on  SwitchB=on  SwitchC=on  SwitchTimes="[1/60  5/60]"  External=on  BreakerResistance=0.01  SnubberResistance=1e6  SnubberCapacitance=inf  Measurements=None
  Voltage Measurement : spsVoltageMeasurementLib/Voltage Measurement  PhasorSimulation=off  OutputType=Complex  PSBequivalent=0
  Zero-Order Hold : ZeroOrderHold  SampleTime=Ts_Control
  Zero-Order Hold1 : ZeroOrderHold  SampleTime=Ts_Control
  Zero-Order Hold2 : ZeroOrderHold  SampleTime=Ts_Control
  A : PMIOPort  Side=Left
  B : PMIOPort  Port=2  Side=Left
  C : PMIOPort  Port=3  Side=Left
  P : PMIOPort  Port=4  Side=Right
  N : PMIOPort  Port=5  Side=Right
  tag scope: PSM3_C=global, PSM3_CRaW=global, PSM3_V=global, PSM3_VRaw=global, PSM4_V3=global
  wires:
  IL2/1 -> [PSM3_CRaW], Zero-Order Hold2/1
  Zero-Order Hold2/1 -> [PSM3_C]
  Zero-Order Hold/1 -> [PSM3_V]
  IL1/1 -> [PSM3_VRaw], Zero-Order Hold/1
  [Breaker3] -> Three-Phase Breaker1/1
  [En_pulses_INV3] -> Logical Operator/2
  Logical Operator/1 -> Inverter1/1
  PWM/1 -> PWM Generator (2-Level)/1
  PWM Generator (2-Level)/1 -> Logical Operator/1
  Voltage Measurement/1 -> Zero-Order Hold1/1
  Zero-Order Hold1/1 -> [PSM4_V3]
  connections:
  IL2/RConn1 -- A/RConn1
  C/RConn1 -- IL2/RConn3
  B/RConn1 -- IL2/RConn2
  IL1/LConn3 -- L1/LConn3
  L1/LConn2 -- IL1/LConn2
  IL1/LConn1 -- L1/LConn1
  IL2/LConn3 -- L2/LConn3
  IL2/LConn2 -- L2/LConn2
  IL2/LConn1 -- L2/LConn1
  Cf/LConn3 -- Neutral1/LConn1 -- Ground/LConn1 -- Cf/LConn1 -- Cf/LConn2
  L2/RConn3 -- Cf/RConn3 -- IL1/RConn3
  L2/RConn2 -- Cf/RConn2 -- IL1/RConn2
  Cf/RConn1 -- IL1/RConn1 -- L2/RConn1
  Three-Phase Breaker1/LConn2 -- L1/RConn2
  L1/RConn1 -- Three-Phase Breaker1/LConn1
  L1/RConn3 -- Three-Phase Breaker1/LConn3
  Inverter1/LConn2 -- Three-Phase Breaker1/RConn2
  Inverter1/LConn3 -- Three-Phase Breaker1/RConn3
  Inverter1/LConn1 -- Three-Phase Breaker1/RConn1
  Voltage Measurement/LConn2 -- N/RConn1 -- Inverter1/RConn2 -- Series RLC Branch/RConn1
  Series RLC Branch/LConn1 -- Inverter1/RConn1 -- P/RConn1 -- Voltage Measurement/LConn1

== system Grid_PBFORCAPF_ab_Detail_2013b_616/Load ==
  Cdc : spsSeriesRLCBranchLib/Series RLC Branch  LConnTagsString=__new0  RConnTagsString=__new0  BranchType=C  Resistance=RL  Inductance=10e-6  SetiL0=off  InitialCurrent=2000  Capacitance=165e-6  Setx0=on  InitialVoltage=500  Measurements=Branch voltage and current
  IL2 : spsThreePhaseVIMeasurementLib/Three-Phase V-I Measurement  VoltageMeasurement=no  SetLabelV=off  LabelV=Vpcc  Vpu=off  VpuLL=off  CurrentMeasurement=yes  SetLabelI=off  LabelI=ILoad  Ipu=off  Pbase=100e6  Vbase=280  OutputType=Complex  PhasorSimulation=off  PSBequivalent=0
  Inverter1 : spsUniversalBridgeLib/Universal Bridge  Arms=3  SnubberResistance=1e5  SnubberCapacitance=inf  Device=Diodes  Ron=1e-3  Lon=0  ForwardVoltages="[  0  0  ]"  ForwardVoltage=0  GTOparameters=[ 10e-6 , 20e-6 ]  IGBTparameters=[ 1e-6 , 2e-6 ]  Measurements=None  Measurements_2=None  converterType=Rectifier
  L1 : spsThreePhaseSeriesRLCBranchLib/Three-Phase Series RLC Branch  LConnTagsString=A|B|C  RConnTagsString=A|B|C  BranchType=RL  Resistance=R2  Inductance=L2_DG1*2  Capacitance=1e-6  Measurements=Branch currents
  L2 : spsThreePhaseSeriesRLCBranchLib/Three-Phase Series RLC Branch  LConnTagsString=A|B|C  RConnTagsString=A|B|C  BranchType=R  Resistance=115  Inductance=L2  Capacitance=1e-6  Measurements=Branch currents
  Neutral1 : spsNeutralLib/Neutral  LConnTagsString=a  NodeNumber=10
      settings: AttributesFormatString=node %<NodeNumber>  SourceProductBaseCode=PS
  RL : spsSeriesRLCBranchLib/Series RLC Branch  LConnTagsString=__new0  RConnTagsString=__new0  BranchType=R  Resistance=115/4  Inductance=10e-6  SetiL0=off  InitialCurrent=2000  Capacitance=17.55e-3  Setx0=on  InitialVoltage=700  Measurements=Branch current
  Three-Phase Breaker1 : spsThreePhaseBreakerLib/Three-Phase Breaker  InitialState=open  SwitchA=on  SwitchB=on  SwitchC=on  SwitchTimes="[1/60  5/60]"  External=on  BreakerResistance=0.01  SnubberResistance=1e6  SnubberCapacitance=inf  Measurements=None
  Three-Phase Breaker2 : spsThreePhaseBreakerLib/Three-Phase Breaker  InitialState=open  SwitchA=on  SwitchB=on  SwitchC=on  SwitchTimes="[1/60  5/60]"  External=on  BreakerResistance=0.01  SnubberResistance=1e6  SnubberCapacitance=inf  Measurements=None
  Zero-Order Hold1 : ZeroOrderHold  SampleTime=Ts_Control
  A : PMIOPort  Side=Left
  B : PMIOPort  Port=2  Side=Left
  C : PMIOPort  Port=3  Side=Left
  tag scope: PSM4_C=global
  wires:
  Zero-Order Hold1/1 -> [PSM4_C]
  IL2/1 -> Zero-Order Hold1/1
  [BreakerNL] -> Three-Phase Breaker1/1
  [BreakerLL] -> Three-Phase Breaker2/1
  connections:
  RL/LConn1 -- Inverter1/RConn2
  IL2/LConn1 -- A/RConn1
  IL2/LConn2 -- B/RConn1
  IL2/LConn3 -- C/RConn1
  Inverter1/RConn1 -- RL/RConn1
  L2/RConn1 -- L2/RConn2 -- L2/RConn3 -- Neutral1/LConn1
  L1/LConn1 -- Inverter1/LConn1
  L1/LConn2 -- Inverter1/LConn2
  L1/LConn3 -- Inverter1/LConn3
  Three-Phase Breaker2/LConn1 -- L2/LConn1
  L2/LConn2 -- Three-Phase Breaker2/LConn2
  L2/LConn3 -- Three-Phase Breaker2/LConn3
  Three-Phase Breaker2/RConn1 -- L1/RConn1 -- IL2/RConn1
  Three-Phase Breaker2/RConn2 -- L1/RConn2 -- IL2/RConn2
  Three-Phase Breaker2/RConn3 -- L1/RConn3 -- IL2/RConn3

== system Grid_PBFORCAPF_ab_Detail_2013b_616/Measure ==
  Add : Sum  Inputs=+-
  CLARKE : Subsystem
  Demux : Demux  Outputs=2
  ICLARKE : Subsystem
  MSOGIs_A : Subsystem  mask{h=[1 5 7 11 13 17 19 23 25], KIh=[1 1 1 1 1 1 1 1 1]*314, Ts=Ts_Control}
      mask prompts: h "Harmonic order"; KIh "Integral gains of SOGI KIh"; Ts "Sampling time"
  MSOGIs_B : Subsystem  mask{h=[1 5 7 11 13 17 19 23 25], KIh=[1 1 1 1 1 1 1 1 1]*314, Ts=Ts_Control}
      mask prompts: h "Harmonic order"; KIh "Integral gains of SOGI KIh"; Ts "Sampling time"
  Mux6 : Mux  Inputs=2
  Product : Product
  Product1 : Product
  Product2 : Product
  Scope : Scope
  Scope1 : Scope
  Scope2 : Scope
  tag scope: ILhrefAB1=global, ILhrefAB2=global, ILhrefAB3=global, ILhrefABC=global
  wires:
  ICLARKE/1(ABC) -> Add/2, Scope1/1, [ILhrefABC]
  Product/1 -> [ILhrefAB1], ICLARKE/1(AB)
  [PSM4_C] -> CLARKE/1(ABC), Add/1, Scope/1
  CLARKE/1(AB) -> Demux/1
  [En_COM1] -> Product/1
  MSOGIs_B/1(Ihref) -> Mux6/2
  Demux/2 -> MSOGIs_B/1(in)
  Demux/1 -> MSOGIs_A/1(in)
  MSOGIs_A/1(Ihref) -> Mux6/1
  [En_COM2] -> Product1/1
  [En_COM3] -> Product2/1
  Mux6/1 -> Product2/2, Product1/2, Product/2
  Product1/1 -> [ILhrefAB2]
  Product2/1 -> [ILhrefAB3]
  Add/1 -> Scope2/1
